simulink model "RCAM_SimulinkModel_MeasurementsIncluded"  (R2022b)
settings: Solver=VariableStepAuto  StartTime=0.0  StopTime=TF  RelTol=1e-3
model workspace (MAT data in the model file):
  op_trim1 = opcond.OperatingReport
  op_trim1.Outputs_(1) = opcond.OutputReport
  op_trim1.Outputs_(1).yspec_ = [0; 0; 0; 0; 0; 0; 0; 0; 0; 0; 0]
  op_trim1.Outputs_(1).Block_ = 'RCAM_SimulinkModel_MeasurementsIncluded/Longitudanal params'
  op_trim1.Outputs_(1).PortWidth_ = 11
  op_trim1.Outputs_(1).PortNumber_ = NaN
  op_trim1.Outputs_(1).y_ = [-0.0703667599908; 0; 0; 85.426778064; 1.7763568394e-15; 0.1; -0.1; -2.07939112262e-17; 2.60928687122e-20; 0; 5.61527919237e-18]
  op_trim1.Outputs_(1).Known_ = [0; 0; 0; 0; 0; 0; 0; 0; 0; 0; 0]
  op_trim1.Outputs_(1).Min_ = [-Inf; -Inf; -Inf; -Inf; -Inf; -Inf; -Inf; -Inf; -Inf; -Inf; -Inf]
  op_trim1.Outputs_(1).Max_ = [Inf; Inf; Inf; Inf; Inf; Inf; Inf; Inf; Inf; Inf; Inf]
  op_trim1.Outputs_(2) = opcond.OutputReport
  op_trim1.Outputs_(2).yspec_ = [0; 0; 0; 0; 0; 0; 0; 0]
  op_trim1.Outputs_(2).Block_ = 'RCAM_SimulinkModel_MeasurementsIncluded/Longitudanal params1'
  op_trim1.Outputs_(2).PortWidth_ = 8
  op_trim1.Outputs_(2).PortNumber_ = NaN
  op_trim1.Outputs_(2).y_ = [1.24164682398e-21; 1.97794051519e-12; 0; 2.79119467282e-11; 4.51754209599e-14; 4.49497059304e-14; -2.22902970453e-18; 5.99560148555e-16]
  op_trim1.Outputs_(2).Known_ = [0; 0; 0; 0; 0; 0; 0; 0]
  op_trim1.Outputs_(2).Min_ = [-Inf; -Inf; -Inf; -Inf; -Inf; -Inf; -Inf; -Inf]
  op_trim1.Outputs_(2).Max_ = [Inf; Inf; Inf; Inf; Inf; Inf; Inf; Inf]
  op_trim1.TerminationString_ = 'Operating point specifications were successfully met.'
  op_trim1.OptimizationOutput_.iterations = 3
  op_trim1.OptimizationOutput_.funcCount = 50
  op_trim1.OptimizationOutput_.lssteplength = 1
  op_trim1.OptimizationOutput_.stepsize = 1.76465360904e-12
  op_trim1.OptimizationOutput_.algorithm = 'active-set'
  op_trim1.OptimizationOutput_.firstorderopt = 0
  op_trim1.OptimizationOutput_.constrviolation = 1.09311670826e-10
  op_trim1.OptimizationOutput_.message = 'Local minimum found that satisfies the constraints.
    | 
    | Optimization completed because the objective function is non-decreasing in 
    | feasible directions, to within the value of the optimality tolerance,
    | and constraints are satisfied to within the  value of the constraint tolerance.
    | 
    | <stopping criteria details>
    | 
    | Optimization completed: The first-order optimality measure, 0.000000e+00, is less
    | than options.OptimalityTolerance = 1.000000e-06, and the maximum constraint violation,
    | 1.093117e-10,is less than options.ConstraintTolerance = 1.000000e-06.'
  op_trim1.OptimizationOutput_.bestfeasible.x = [3.83990855256e-12; -8.52844712726; 1.24164682398e-21; -0.0703667599908; 1.97794051519e-12; 2.79119467282e-11; 4.51754209599e-14; 5.61527919237e-18; 5.99560148555e-16; 0; -1.68425367217e-11; 0.0570564846138; -4.45835422921e-11; -0.00660921864732; -0.00660921862469]
  op_trim1.OptimizationOutput_.bestfeasible.fval = 0
  op_trim1.OptimizationOutput_.bestfeasible.constrviolation = 1.09311670826e-10
  op_trim1.OptimizationOutput_.bestfeasible.firstorderopt = 0
  op_trim1.OptimizationOutput_.progress = {'<font face="monospaced"; size=3><BR>', 'Optimizing to solve for all desired dx/dt=0, x(k+1)-x(k)=0, and y=ydes.<BR>', ' <BR>', '(Maximum Error)  Block<BR>', ' ---------------------------------------------------------<BR>', '(8.48584e+00) RCAM_SimulinkModel_MeasurementsIncluded/Subsystem/Integrator1<BR>', '(6.74979e-02) RCAM_SimulinkModel_MeasurementsIncluded/Subsystem/Integrator<BR>', '(1.09312e-10) RCAM_SimulinkModel_MeasurementsIncluded/Subsystem/Integrator<BR>', '(1.09312e-10) RCAM_SimulinkModel_MeasurementsIncluded/Subsystem/Integrator<BR>', ' <BR>', 'Operating point specifications were successfully met.<BR>'}
  op_trim1.Model_ = 'RCAM_SimulinkModel_MeasurementsIncluded'
  op_trim1.States_(1) = opcond.StateReport
  op_trim1.States_(1).dx_ = [-1.79150641595; -9.84145888603e-21; -1.09311670826e-10; -1.12011192723e-15; -2.36517128845e-12; -8.48652118189e-17; 1.39136811521e-15; -0.0703667599908; 1.39368852664e-14]
  op_trim1.States_(1).Nx_ = 9
  op_trim1.States_(1).Block_ = 'RCAM_SimulinkModel_MeasurementsIncluded/Subsystem/Integrator'
  op_trim1.States_(1).x_ = [85; 3.83990855256e-12; -8.52844712726; 1.24164682398e-21; -0.0703667599908; 1.97794051519e-12; 2.79119467282e-11; 0.1; 4.51754209599e-14]
  op_trim1.States_(1).SteadyState_ = [0; 1; 1; 1; 1; 1; 1; 0; 1]
  op_trim1.States_(1).dxMin_ = [-Inf; -Inf; -Inf; -Inf; -Inf; -Inf; -Inf; -Inf; -Inf]
  op_trim1.States_(1).dxMax_ = [Inf; Inf; Inf; Inf; Inf; Inf; Inf; Inf; Inf]
  op_trim1.States_(1).Known_ = [1; 0; 0; 0; 0; 0; 0; 1; 0]
  op_trim1.States_(1).Min_ = [-Inf; -Inf; -Inf; -Inf; -Inf; -Inf; -Inf; -Inf; -Inf]
  op_trim1.States_(1).Max_ = [Inf; Inf; Inf; Inf; Inf; Inf; Inf; Inf; Inf]
  op_trim1.States_(2) = opcond.StateReport
  op_trim1.States_(2).dx_ = [85.426778064; -2.22902970453e-18; 1.7763568394e-15]
  op_trim1.States_(2).Nx_ = 3
  op_trim1.States_(2).Block_ = 'RCAM_SimulinkModel_MeasurementsIncluded/Subsystem/Integrator1'
  op_trim1.States_(2).x_ = [5.61527919237e-18; 5.99560148555e-16; 0]
  op_trim1.States_(2).SteadyState_ = [0; 1; 1]
  op_trim1.States_(2).dxMin_ = [-Inf; -Inf; -Inf]
  op_trim1.States_(2).dxMax_ = [Inf; Inf; Inf]
  op_trim1.States_(2).Known_ = [0; 0; 0]
  op_trim1.States_(2).Min_ = [-Inf; -Inf; -Inf]
  op_trim1.States_(2).Max_ = [Inf; Inf; Inf]
  op_trim1.Inputs_ = opcond.InputReport
  op_trim1.Inputs_.Block_ = 'RCAM_SimulinkModel_MeasurementsIncluded/control inputs (5x1)'
  op_trim1.Inputs_.PortWidth_ = 5
  op_trim1.Inputs_.PortDimensions_ = [1 5]
  op_trim1.Inputs_.u_ = [-1.68425367217e-11; 0.0570564846138; -4.45835422921e-11; -0.00660921864732; -0.00660921862469]
  op_trim1.Inputs_.Known_ = [0; 0; 0; 0; 0]
  op_trim1.Inputs_.Min_ = [-Inf; -Inf; -Inf; -Inf; -Inf]
  op_trim1.Inputs_.Max_ = [Inf; Inf; Inf; Inf; Inf]
  op_trim4 = opcond.OperatingReport
  op_trim4.Outputs_(1) = opcond.OutputReport
  op_trim4.Outputs_(1).yspec_ = 0
  op_trim4.Outputs_(1).Block_ = 'RCAM_SimulinkModel_MeasurementsIncluded/Out1'
  op_trim4.Outputs_(1).PortWidth_ = 1
  op_trim4.Outputs_(1).PortNumber_ = NaN
  op_trim4.Outputs_(1).y_ = -8.89207430366e-22
  op_trim4.Outputs_(1).Known_ = 0
  op_trim4.Outputs_(1).Min_ = -Inf
  op_trim4.Outputs_(1).Max_ = Inf
  op_trim4.Outputs_(2) = opcond.OutputReport
  op_trim4.Outputs_(2).yspec_ = 0
  op_trim4.Outputs_(2).Block_ = 'RCAM_SimulinkModel_MeasurementsIncluded/Out2'
  op_trim4.Outputs_(2).PortWidth_ = 1
  op_trim4.Outputs_(2).PortNumber_ = NaN
  op_trim4.Outputs_(2).Known_ = 0
  op_trim4.Outputs_(2).Min_ = -Inf
  op_trim4.Outputs_(2).Max_ = Inf
  op_trim4.Outputs_(3) = opcond.OutputReport
  op_trim4.Outputs_(3).yspec_ = 0
  op_trim4.Outputs_(3).Block_ = 'RCAM_SimulinkModel_MeasurementsIncluded/Out3'
  op_trim4.Outputs_(3).PortWidth_ = 1
  op_trim4.Outputs_(3).PortNumber_ = NaN
  op_trim4.Outputs_(3).y_ = 0
  op_trim4.Outputs_(3).Known_ = 0
  op_trim4.Outputs_(3).Min_ = -Inf
  op_trim4.Outputs_(3).Max_ = Inf
  op_trim4.Outputs_(4) = opcond.OutputReport
  op_trim4.Outputs_(4).yspec_ = 0
  op_trim4.Outputs_(4).Block_ = 'RCAM_SimulinkModel_MeasurementsIncluded/Out4'
  op_trim4.Outputs_(4).PortWidth_ = 1
  op_trim4.Outputs_(4).PortNumber_ = NaN
  op_trim4.Outputs_(4).y_ = 303.599941428
  op_trim4.Outputs_(4).Known_ = 0
  op_trim4.Outputs_(4).Min_ = -Inf
  op_trim4.Outputs_(4).Max_ = Inf
  op_trim4.Outputs_(5) = opcond.OutputReport
  op_trim4.Outputs_(5).yspec_ = 0
  op_trim4.Outputs_(5).Block_ = 'RCAM_SimulinkModel_MeasurementsIncluded/Out5'
  op_trim4.Outputs_(5).PortWidth_ = 1
  op_trim4.Outputs_(5).PortNumber_ = NaN
  op_trim4.Outputs_(5).y_ = 2.84217094304e-14
  op_trim4.Outputs_(5).Known_ = 0
  op_trim4.Outputs_(5).Min_ = -Inf
  op_trim4.Outputs_(5).Max_ = Inf
  op_trim4.Outputs_(6) = opcond.OutputReport
  op_trim4.Outputs_(6).yspec_ = 0
  op_trim4.Outputs_(6).Block_ = 'RCAM_SimulinkModel_MeasurementsIncluded/Out6'
  op_trim4.Outputs_(6).PortWidth_ = 1
  op_trim4.Outputs_(6).PortNumber_ = NaN
  op_trim4.Outputs_(6).y_ = 0.154149438561
  op_trim4.Outputs_(6).Known_ = 0
  op_trim4.Outputs_(6).Min_ = -Inf
  op_trim4.Outputs_(6).Max_ = Inf
  op_trim4.Outputs_(7) = opcond.OutputReport
  op_trim4.Outputs_(7).yspec_ = 0
  op_trim4.Outputs_(7).Block_ = 'RCAM_SimulinkModel_MeasurementsIncluded/Out7'
  op_trim4.Outputs_(7).PortWidth_ = 1
  op_trim4.Outputs_(7).PortNumber_ = NaN
  op_trim4.Outputs_(7).y_ = -0.154149438561
  op_trim4.Outputs_(7).Known_ = 0
  op_trim4.Outputs_(7).Min_ = -Inf
  op_trim4.Outputs_(7).Max_ = Inf
  op_trim4.Outputs_(8) = opcond.OutputReport
  op_trim4.Outputs_(8).yspec_ = 0
  op_trim4.Outputs_(8).Block_ = 'RCAM_SimulinkModel_MeasurementsIncluded/Out8'
  op_trim4.Outputs_(8).PortWidth_ = 1
  op_trim4.Outputs_(8).PortNumber_ = NaN
  op_trim4.Outputs_(8).y_ = -9.36156617709e-17
  op_trim4.Outputs_(8).Known_ = 0
  op_trim4.Outputs_(8).Min_ = -Inf
  op_trim4.Outputs_(8).Max_ = Inf
  op_trim4.Outputs_(9) = opcond.OutputReport
  op_trim4.Outputs_(9).yspec_ = 0
  op_trim4.Outputs_(9).Block_ = 'RCAM_SimulinkModel_MeasurementsIncluded/Out9'
  op_trim4.Outputs_(9).PortWidth_ = 1
  op_trim4.Outputs_(9).PortNumber_ = NaN
  op_trim4.Outputs_(9).y_ = 1.82219532413e-23
  op_trim4.Outputs_(9).Known_ = 0
  op_trim4.Outputs_(9).Min_ = -Inf
  op_trim4.Outputs_(9).Max_ = Inf
  op_trim4.Outputs_(10) = opcond.OutputReport
  op_trim4.Outputs_(10).yspec_ = 0
  op_trim4.Outputs_(10).Block_ = 'RCAM_SimulinkModel_MeasurementsIncluded/Out10'
  op_trim4.Outputs_(10).PortWidth_ = 1
  op_trim4.Outputs_(10).PortNumber_ = NaN
  op_trim4.Outputs_(10).y_ = 2000
  op_trim4.Outputs_(10).Known_ = 0
  op_trim4.Outputs_(10).Min_ = -Inf
  op_trim4.Outputs_(10).Max_ = Inf
  op_trim4.Outputs_(11) = opcond.OutputReport
  op_trim4.Outputs_(11).yspec_ = 0
  op_trim4.Outputs_(11).Block_ = 'RCAM_SimulinkModel_MeasurementsIncluded/Out11'
  op_trim4.Outputs_(11).PortWidth_ = 1
  op_trim4.Outputs_(11).PortNumber_ = NaN
  op_trim4.Outputs_(11).y_ = -4.81206016551e-15
  op_trim4.Outputs_(11).Known_ = 0
  op_trim4.Outputs_(11).Min_ = -Inf
  op_trim4.Outputs_(11).Max_ = Inf
  op_trim4.Outputs_(12) = opcond.OutputReport
  op_trim4.Outputs_(12).yspec_ = 0
  op_trim4.Outputs_(12).Block_ = 'RCAM_SimulinkModel_MeasurementsIncluded/Out12'
  op_trim4.Outputs_(12).PortWidth_ = 1
  op_trim4.Outputs_(12).PortNumber_ = NaN
  op_trim4.Outputs_(12).y_ = -1.12785253339e-29
  op_trim4.Outputs_(12).Known_ = 0
  op_trim4.Outputs_(12).Min_ = -Inf
  op_trim4.Outputs_(12).Max_ = Inf
  op_trim4.Outputs_(13) = opcond.OutputReport
  op_trim4.Outputs_(13).yspec_ = 0
  op_trim4.Outputs_(13).Block_ = 'RCAM_SimulinkModel_MeasurementsIncluded/Out13'
  op_trim4.Outputs_(13).PortWidth_ = 1
  op_trim4.Outputs_(13).PortNumber_ = NaN
  op_trim4.Outputs_(13).y_ = 2.25303334092e-30
  op_trim4.Outputs_(13).Known_ = 0
  op_trim4.Outputs_(13).Min_ = -Inf
  op_trim4.Outputs_(13).Max_ = Inf
  op_trim4.Outputs_(14) = opcond.OutputReport
  op_trim4.Outputs_(14).yspec_ = 0
  op_trim4.Outputs_(14).Block_ = 'RCAM_SimulinkModel_MeasurementsIncluded/Out14'
  op_trim4.Outputs_(14).PortWidth_ = 1
  op_trim4.Outputs_(14).PortNumber_ = NaN
  op_trim4.Outputs_(14).Known_ = 0
  op_trim4.Outputs_(14).Min_ = -Inf
  op_trim4.Outputs_(14).Max_ = Inf
  op_trim4.Outputs_(15) = opcond.OutputReport
  op_trim4.Outputs_(15).yspec_ = 0
  op_trim4.Outputs_(15).Block_ = 'RCAM_SimulinkModel_MeasurementsIncluded/Out15'
  op_trim4.Outputs_(15).PortWidth_ = 1
  op_trim4.Outputs_(15).PortNumber_ = NaN
  op_trim4.Outputs_(15).y_ = 3.13092287559e-10
  op_trim4.Outputs_(15).Known_ = 0
  op_trim4.Outputs_(15).Min_ = -Inf
  op_trim4.Outputs_(15).Max_ = Inf
  op_trim4.Outputs_(16) = opcond.OutputReport
  op_trim4.Outputs_(16).yspec_ = 0
  op_trim4.Outputs_(16).Block_ = 'RCAM_SimulinkModel_MeasurementsIncluded/Out16'
  op_trim4.Outputs_(16).PortWidth_ = 1
  op_trim4.Outputs_(16).PortNumber_ = NaN
  op_trim4.Outputs_(16).y_ = 2.6300151694e-11
  op_trim4.Outputs_(16).Known_ = 0
  op_trim4.Outputs_(16).Min_ = -Inf
  op_trim4.Outputs_(16).Max_ = Inf
  op_trim4.Outputs_(17) = opcond.OutputReport
  op_trim4.Outputs_(17).yspec_ = 0
  op_trim4.Outputs_(17).Block_ = 'RCAM_SimulinkModel_MeasurementsIncluded/Out17'
  op_trim4.Outputs_(17).PortWidth_ = 1
  op_trim4.Outputs_(17).PortNumber_ = NaN
  op_trim4.Outputs_(17).y_ = 2.59882972015e-11
  op_trim4.Outputs_(17).Known_ = 0
  op_trim4.Outputs_(17).Min_ = -Inf
  op_trim4.Outputs_(17).Max_ = Inf
  op_trim4.Outputs_(18) = opcond.OutputReport
  op_trim4.Outputs_(18).yspec_ = 0
  op_trim4.Outputs_(18).Block_ = 'RCAM_SimulinkModel_MeasurementsIncluded/Out18'
  op_trim4.Outputs_(18).PortWidth_ = 1
  op_trim4.Outputs_(18).PortNumber_ = NaN
  op_trim4.Outputs_(18).y_ = -5.53218393675e-21
  op_trim4.Outputs_(18).Known_ = 0
  op_trim4.Outputs_(18).Min_ = -Inf
  op_trim4.Outputs_(18).Max_ = Inf
  op_trim4.Outputs_(19) = opcond.OutputReport
  op_trim4.Outputs_(19).yspec_ = 0
  op_trim4.Outputs_(19).Block_ = 'RCAM_SimulinkModel_MeasurementsIncluded/Out19'
  op_trim4.Outputs_(19).PortWidth_ = 1
  op_trim4.Outputs_(19).PortNumber_ = NaN
  op_trim4.Outputs_(19).y_ = -3.37584985413e-15
  op_trim4.Outputs_(19).Known_ = 0
  op_trim4.Outputs_(19).Min_ = -Inf
  op_trim4.Outputs_(19).Max_ = Inf
  op_trim4.TerminationString_ = 'Operating point specifications were successfully met.'
  op_trim4.OptimizationOutput_.iterations = 5
  op_trim4.OptimizationOutput_.funcCount = 89
  op_trim4.OptimizationOutput_.lssteplength = 1
  op_trim4.OptimizationOutput_.stepsize = 6.09988133806e-14
  op_trim4.OptimizationOutput_.algorithm = 'active-set'
  op_trim4.OptimizationOutput_.firstorderopt = 0
  op_trim4.OptimizationOutput_.constrviolation = 2.77456783783e-13
  op_trim4.OptimizationOutput_.message = 'Local minimum found that satisfies the constraints.
    | 
    | Optimization completed because the objective function is non-decreasing in 
    | feasible directions, to within the value of the optimality tolerance,
    | and constraints are satisfied to within the  value of the constraint tolerance.
    | 
    | <stopping criteria details>
    | 
    | Optimization completed: The first-order optimality measure, 0.000000e+00, is less
    | than options.OptimalityTolerance = 1.000000e-06, and the maximum constraint violation,
    | 2.774568e-13,is less than options.ConstraintTolerance = 1.000000e-06.'
  op_trim4.OptimizationOutput_.bestfeasible.x = [7.8900455082e-09; -46.6146375634; -1.12785253339e-29; -8.89207430366e-22; 2.25303334092e-30; 3.13092287559e-10; 0.154149438561; 2.6300151694e-11; -4.81206016551e-15; -3.37584985413e-15; -2000; -3.91547360029e-11; 0.0622828487863; 6.9872549314e-11; -17.5996827056; -17.5996827055]
  op_trim4.OptimizationOutput_.bestfeasible.fval = 0
  op_trim4.OptimizationOutput_.bestfeasible.constrviolation = 2.77456783783e-13
  op_trim4.OptimizationOutput_.bestfeasible.firstorderopt = 0
  op_trim4.OptimizationOutput_.progress = {'<font face="monospaced"; size=3><BR>', 'Optimizing to solve for all desired dx/dt=0, x(k+1)-x(k)=0, and y=ydes.<BR>', ' <BR>', '(Maximum Error)  Block<BR>', ' ---------------------------------------------------------<BR>', '(1.13552e+02) RCAM_SimulinkModel_MeasurementsIncluded/Subsystem/Integrator<BR>', '(1.15667e+01) RCAM_SimulinkModel_MeasurementsIncluded/Subsystem/Integrator<BR>', '(1.33781e-01) RCAM_SimulinkModel_MeasurementsIncluded/Subsystem/Integrator<BR>', '(1.01514e-05) RCAM_SimulinkModel_MeasurementsIncluded/Subsystem/Integrator<BR>', '(2.77457e-13) RCAM_SimulinkModel_MeasurementsIncluded/Subsystem/Integrator<BR>', '(2.77457e-13) RCAM_SimulinkModel_MeasurementsIncluded/Subsystem/Integrator<BR>', ' <BR>', 'Operating point specifications were successfully met.<BR>'}
  op_trim4.Model_ = 'RCAM_SimulinkModel_MeasurementsIncluded'
  op_trim4.States_(1) = opcond.StateReport
  op_trim4.States_(1).dx_ = [-19.2593254017; -5.96312696523e-23; -2.77456783783e-13; 4.37729600243e-24; -6.0210444038e-14; 2.42390872438e-23; -1.09717032286e-29; -8.89207430366e-22; 1.99832451914e-30]
  op_trim4.States_(1).Nx_ = 9
  op_trim4.States_(1).Block_ = 'RCAM_SimulinkModel_MeasurementsIncluded/Subsystem/Integrator'
  op_trim4.States_(1).x_ = [300; 7.8900455082e-09; -46.6146375634; -1.12785253339e-29; -8.89207430366e-22; 2.25303334092e-30; 3.13092287559e-10; 0.154149438561; 2.6300151694e-11]
  op_trim4.States_(1).SteadyState_ = [0; 1; 1; 1; 1; 1; 1; 1; 1]
  op_trim4.States_(1).dxMin_ = [-Inf; -Inf; -Inf; -Inf; -Inf; -Inf; -Inf; -Inf; -Inf]
  op_trim4.States_(1).dxMax_ = [Inf; Inf; Inf; Inf; Inf; Inf; Inf; Inf; Inf]
  op_trim4.States_(1).Known_ = [1; 0; 0; 0; 0; 0; 0; 0; 0]
  op_trim4.States_(1).Min_ = [-Inf; -Inf; -Inf; -Inf; -Inf; -Inf; -Inf; -Inf; -Inf]
  op_trim4.States_(1).Max_ = [Inf; Inf; Inf; Inf; Inf; Inf; Inf; Inf; Inf]
  op_trim4.States_(2) = opcond.StateReport
  op_trim4.States_(2).dx_ = [303.599941428; -5.53218393675e-21; 2.84217094304e-14]
  op_trim4.States_(2).Nx_ = 3
  op_trim4.States_(2).Block_ = 'RCAM_SimulinkModel_MeasurementsIncluded/Subsystem/Integrator1'
  op_trim4.States_(2).x_ = [-4.81206016551e-15; -3.37584985413e-15; -2000]
  op_trim4.States_(2).SteadyState_ = [0; 1; 1]
  op_trim4.States_(2).dxMin_ = [-Inf; -Inf; -Inf]
  op_trim4.States_(2).dxMax_ = [Inf; Inf; Inf]
  op_trim4.States_(2).Known_ = [0; 0; 0]
  op_trim4.States_(2).Min_ = [-Inf; -Inf; -Inf]
  op_trim4.States_(2).Max_ = [Inf; Inf; Inf]
  op_trim4.Inputs_ = opcond.InputReport
  op_trim4.Inputs_.Block_ = 'RCAM_SimulinkModel_MeasurementsIncluded/control inputs (5x1)'
  op_trim4.Inputs_.PortWidth_ = 5
  op_trim4.Inputs_.PortDimensions_ = [1 5]
  op_trim4.Inputs_.u_ = [-3.91547360029e-11; 0.0622828487863; 6.9872549314e-11; -17.5996827056; -17.5996827055]
  op_trim4.Inputs_.Known_ = [0; 0; 0; 0; 0]
  op_trim4.Inputs_.Min_ = [-Inf; -Inf; -Inf; -Inf; -Inf]
  op_trim4.Inputs_.Max_ = [Inf; Inf; Inf; Inf; Inf]
values from neighbouring files (symbols this model uses):
  X0 = [100 ... (first row only)    [RCAM_model_initialConditions.m]    (also in designPIL.m = [85)
  XYZ0 = [0;0;0]    [RCAM_model_initialConditions.m]    (also in designPIL.m)
undefined symbols (not defined in the file or in its folder): RCAM_model
libraries: sharedtransform x1
settings Model: Creator=bendr  LastModifiedBy=bendr
settings DataIOCC: ExternalInput=getinputstruct(op_trim4)  InitialState=getstatestruct(op_trim4)  LoadExternalInput=on  LoadInitialState=on

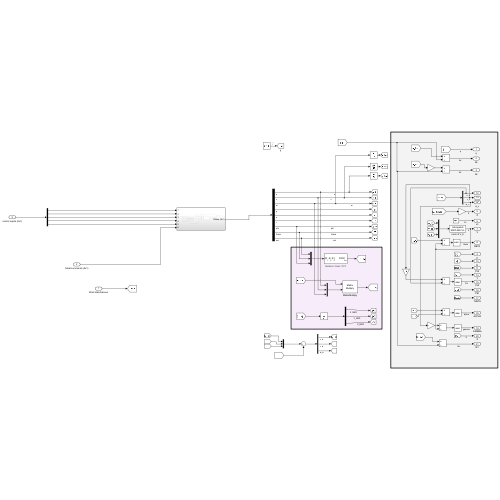
[thumbnail: Simulink's stored preview of the top-level diagram]
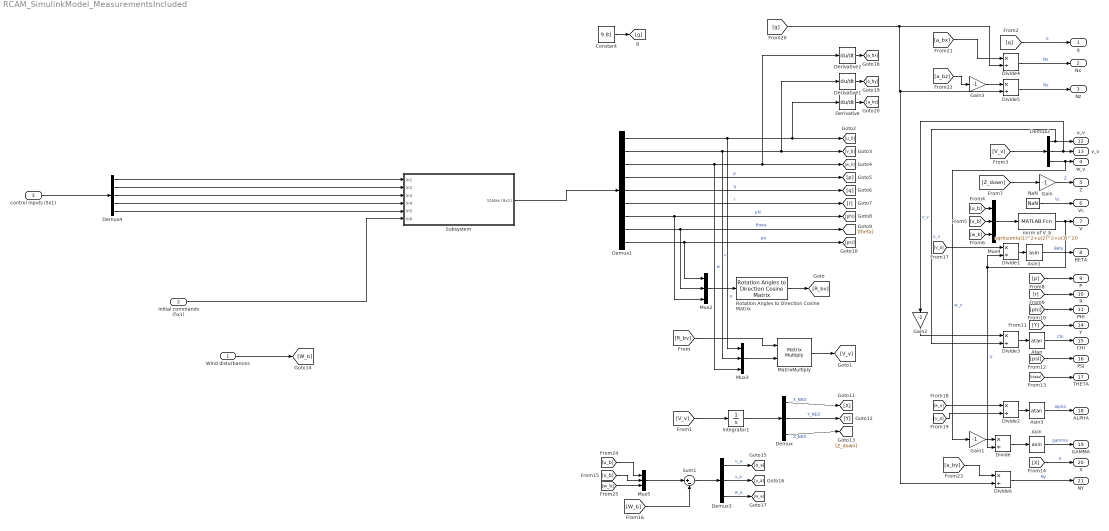
== system RCAM_SimulinkModel_MeasurementsIncluded ==
  Wind disturbances : Inport
  Initial commands (5x1) : Inport  Port=2
  control inputs (5x1) : Inport  Port=3
  Asin : Trigonometry  Operator=asin
  Asin1 : Trigonometry  Operator=asin
  Asin3 : Trigonometry  Operator=atan
  Atan : Trigonometry  Operator=atan
  Constant : Constant  Value=9.81
  Demux : Demux  Outputs=3
  Demux1 : Demux  Outputs=9
  Demux2 : Demux  Outputs=3
  Demux3 : Demux  Outputs=3
  Demux4 : Demux  Outputs=5
  Derivative : Derivative
  Derivative1 : Derivative
  Derivative2 : Derivative
  Divide{,1..6} (7 alike) : Product  Inputs=*/
  Gain{,1..3} (4 alike) : Gain  Gain=-1
  Integrator1 : Integrator  InitialCondition=XYZ0
  MatrixMultiply : Product  Multiplication=Matrix(*)
  Mux{2..5} (4 alike) : Mux  Inputs=3
  NaN : Constant  Value=NaN  OutDataTypeStr=Inherit: Inherit via back propagation
  Rotation Angles to Direction Cosine Matrix : sharedtransform/Rotation Angles to Direction Cosine Matrix  rotationOrder=ZYX  aMode=aMode
  Subsystem : Subsystem
  Sum1 : Sum  Inputs=|+-
  norm of V_b : MATLABFcn  MATLABFcn=sqrt(sum(u(1)^2+u(2)^2+u(3)^2))
  q : Outport
  Nx : Outport  Port=2
  Nz : Outport  Port=3
  w_v : Outport  Port=4
  Z : Outport  Port=5
  Vc : Outport  Port=6
  V : Outport  Port=7
  BETA : Outport  Port=8
  P : Outport  Port=9
  R : Outport  Port=10
  PHI : Outport  Port=11
  u_v : Outport  Port=12
  v_v : Outport  Port=13
  Y : Outport  Port=14
  CHI : Outport  Port=15
  PSI : Outport  Port=16
  THETA : Outport  Port=17
  ALPHA : Outport  Port=18
  GAMMA : Outport  Port=19
  X : Outport  Port=20
  NY : Outport  Port=21
  wires:
  MatrixMultiply/1 -> [V_v]
  [Z_down] -> Gain/1
  Derivative2/1 -> [a_bx]
  [u_b] -> Mux5/1
  [a_bz] -> Gain3/1
  Divide4/1 -> Nx/1  "Nx"
  [v_b] -> Mux5/2
  Asin3/1 -> ALPHA/1  "alpha"
  [psi] -> PSI/1
  [w_a] -> Divide2/1
  [W_b] -> Sum1/2
  Mux5/1 -> Sum1/1
  [u_b] -> Mux4/1
  Demux3/1 -> [u_a]  "u_a"
  Gain3/1 -> Divide5/1
  [a_by] -> Divide6/1
  [a_bx] -> Divide4/1
  [Y] -> Y/1
  Derivative1/1 -> [a_by]
  [w_b] -> Mux5/3
  Mux3/1 -> MatrixMultiply/2
  Asin1/1 -> BETA/1  "Beta"
  Atan/1 -> CHI/1  "Chi"
  Gain2/1 -> Divide3/1
  Constant/1 -> [g]
  Divide3/1 -> Atan/1
  [g] -> Divide4/2, Divide6/2, Divide5/2
  [u_a] -> Divide2/2
  Demux2/1 -> Divide3/2, u_v/1  "u_v"
  Divide2/1 -> Asin3/1
  Integrator1/1 -> Demux/1
  [X] -> X/1  "X"
  Divide/1 -> Asin/1
  Divide1/1 -> Asin1/1
  Sum1/1 -> Demux3/1
  Divide5/1 -> Nz/1  "Nz"
  Gain1/1 -> Divide/1
  Demux3/3 -> [w_a]  "w_a"
  [v_a] -> Divide1/1
  Demux3/2 -> [v_a]  "v_a"
  [p] -> P/1
  Demux1/6 -> [r]  "r"
  Demux2/3 -> Gain1/1, w_v/1  "w_v"
  norm of V_b/1 -> Divide/2, Divide1/2, V/1  "V"
  Wind disturbances/1 -> [W_b]
  [phi] -> PHI/1
  [v_b] -> Mux4/2
  Divide6/1 -> NY/1  "Ny"
  Rotation Angles to Direction Cosine Matrix/1 -> [R_bv]
  [V_v] -> Demux2/1
  Asin/1 -> GAMMA/1  "gamma"
  NaN/1 -> Vc/1  "Vc"
  Demux1/3 -> Mux3/3, Derivative2/1, [w_b]  "w"
  [V_v] -> Integrator1/1
  Demux/1 -> [X]  "X_NED"
  Gain/1 -> Z/1  "Z"
  [R_bv] -> MatrixMultiply/1
  Mux2/1 -> Rotation Angles to Direction Cosine Matrix/1
  [r] -> R/1
  Demux1/2 -> Mux3/2, Derivative1/1, [v_b]  "v"
  Mux4/1 -> norm of V_b/1
  [w_b] -> Mux4/3
  Demux1/4 -> [p]  "p"
  Demux1/1 -> Mux3/1, Derivative/1, [u_b]  "u"
  Demux1/8 -> Mux2/2, [theta]  "theta"
  Demux1/9 -> Mux2/1, [psi]  "psi"
  Demux2/2 -> v_v/1, Gain2/1  "v_v"
  Demux/3 -> [Z_down]  "Z_NED"
  Demux/2 -> [Y]  "Y_NED"
  [q] -> q/1  "q"
  Demux1/7 -> Mux2/3, [phi]  "phi"
  Demux1/5 -> [q]  "q"
  Derivative/1 -> [a_bz]
  [theta] -> THETA/1
  Initial commands (5x1)/1 -> Subsystem/6(In6)
  Subsystem/1(States (9x1)) -> Demux1/1
  Demux4/5 -> Subsystem/5(In5)
  Demux4/3 -> Subsystem/3(In3)
  control inputs (5x1)/1 -> Demux4/1
  Demux4/4 -> Subsystem/4(In4)
  Demux4/2 -> Subsystem/2(In2)
  Demux4/1 -> Subsystem/1(In1)

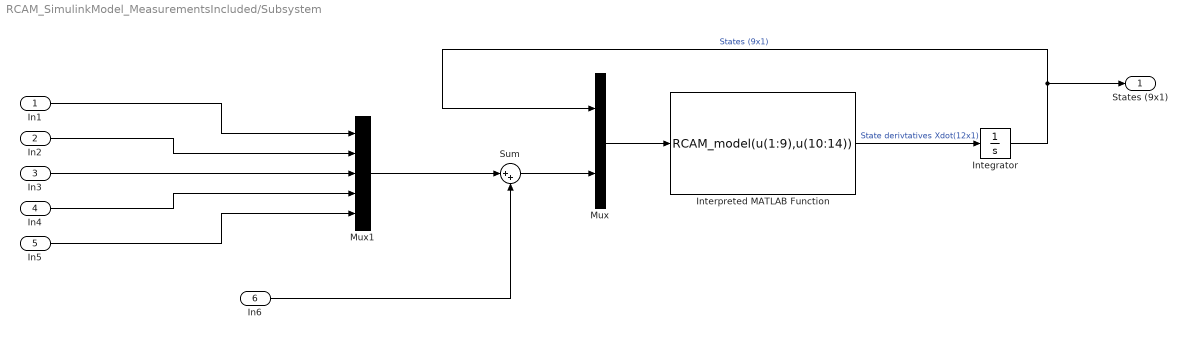
== system RCAM_SimulinkModel_MeasurementsIncluded/Subsystem ==
  In1 : Inport
  In2 : Inport  Port=2
  In3 : Inport  Port=3
  In4 : Inport  Port=4
  In5 : Inport  Port=5
  In6 : Inport  Port=6
  Integrator : Integrator  InitialCondition=X0
  Interpreted MATLAB Function : MATLABFcn  MATLABFcn=RCAM_model(u(1:9),u(10:14))
  Mux : Mux  Inputs=2
  Mux1 : Mux  Inputs=5
  Sum : Sum  Inputs=|++
  States (9x1) : Outport
  wires:
  Mux/1 -> Interpreted MATLAB Function/1
  Integrator/1 -> States (9x1)/1, Mux/1  "States (9x1)"
  Interpreted MATLAB Function/1 -> Integrator/1  "State derivtatives Xdot(12x1)"
  In6/1 -> Sum/2
  Mux1/1 -> Sum/1
  Sum/1 -> Mux/2
  In1/1 -> Mux1/1
  In4/1 -> Mux1/4
  In5/1 -> Mux1/5
  In2/1 -> Mux1/2
  In3/1 -> Mux1/3
